simulink model "AGcontrolPIDvelocidadConObsIntegrador_trapPosFinal2017"  (R2017a)
settings: Solver=ode45  StartTime=0.0  StopTime=20  MaxStep=1e-4  RelTol=1e-5  EnableMultiTasking=on
values from neighbouring files (symbols this model uses):
  alfa_cu = 3.9*10^-3    (= 0.0039)    [InicializaYconstantes.m]
  b_m = bm+(bl/r^2)    (= 1.5e-05)    [InicializaYconstantes.m]
  Cts = 1.091    [InicializaYconstantes.m]
  J_m = Jm+(Jl/r^2)    (= 5.65099476805e-06)    [InicializaYconstantes.m]
  Kd = J_m*n*wpos    (= 0.0113019895361)    [InicializaYconstantes.m]
  Ke_int = 3.2768e10    (= 32768000000)    [InicializaYconstantes.m]
  Ketita_corr = 8000    [InicializaYconstantes.m]
  Kew_corr = 25600e3    (= 25600000)    [InicializaYconstantes.m]
  Ki = J_m*wpos^3    (= 2893.30932124)    [InicializaYconstantes.m]
  Kp = J_m*n*wpos^2    (= 9.04159162887)    [InicializaYconstantes.m]
  lambda = 0.01546    [InicializaYconstantes.m]
  Ld = 6.6*10^-3    (= 0.0066)    [InicializaYconstantes.m]
  Lq = 5.8*10^-3    (= 0.0058)    [InicializaYconstantes.m]
  Pp = 3    [InicializaYconstantes.m]
  r = 314.3008    [InicializaYconstantes.m]
  R1 = -p1i*Lq    (= 29)    [InicializaYconstantes.m]
  R2 = -p1i*Ld    (= 33)    [InicializaYconstantes.m]
  Rs = 1.02    [InicializaYconstantes.m]
  Rs_cero = 1.02    [InicializaYconstantes.m]
  Rts = 55    [InicializaYconstantes.m]
  T_l = Tl/r    (= 0.00499521477515)    [InicializaYconstantes.m]
  Ta = 40    [InicializaYconstantes.m]
  Ts0 = 40    [InicializaYconstantes.m]
undefined symbols (not defined in the file or in its folder): sigbuilder_block
libraries: simulink x1
settings Model: Creator=usuario  LastModifiedBy=usuario
settings DataIOCC: LimitDataPoints=on  SaveFormat=Array
settings OptimizationCC: ExpressionDepthLimit=2147483647  LifeSpan=inf
settings DebuggingCC: UnderspecifiedInitializationDetection=Classic  MergeDetectMultiDrivingBlocksExec=none  SolverPrmCheckMsg=warning  StateNameClashWarn=warning  SFUnexpectedBacktrackingDiag=warning  SFNoUnconditionalDefaultTransitionDiag=warning  SFExecutionAtInitializationDiag=none
settings HardwareCC: ProdBitPerPointer=32  ProdBitPerSizeT=32  ProdBitPerPtrDiffT=32  ProdLargestAtomicFloat=None  ProdIntDivRoundTo=Undefined  ProdEndianess=Unspecified  ProdWordSize=32  ProdHWDeviceType=32-bit Generic
settings ModelReferenceCC: PropagateSignalLabelsOutOfModel=off
settings GRTTargetCC: TargetLangStandard=C89/C90 (ANSI)  GeneratePreprocessorConditionals=Disable all
settings ConfigComp: CovMetricSettings=dw  CovHtmlReporting=on  CovSaveCumulativeToWorkspaceVar=on  CovSaveSingleToWorkspaceVar=on  CovExternalEMLEnable=off

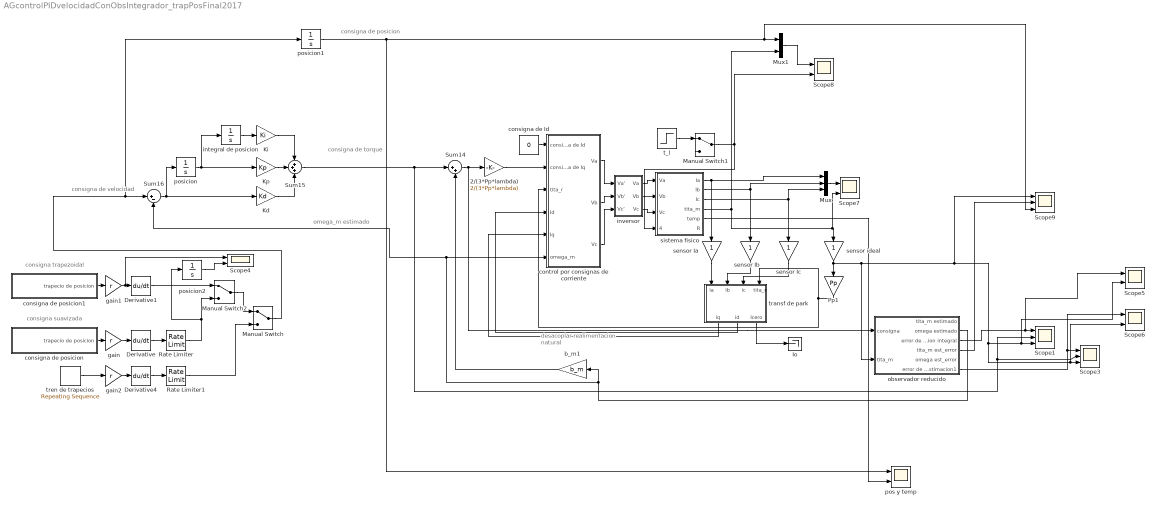
== system AGcontrolPIDvelocidadConObsIntegrador_trapPosFinal2017 ==
  note: consigna trapezoidal
  note: consigna suavizada
  note: consigna de posicion
  note: consigna de velocidad
  note: omega_m estimado
  note: consigna
      | de torque
  note: desacoplar
      | realimentacion natural
  " control por consignas de corriente" : Subsystem
  " pos y temp" : Scope  NumInputPorts=2
  2/(3*Pp*lambda) : Gain  Gain=2/(3*Pp*lambda)
  Derivative : Derivative
  Derivative1 : Derivative
  Derivative4 : Derivative
  Io : Terminator
  Kd : Gain  Gain=Kd
  Ki : Gain  Gain=Ki
  Kp : Gain  Gain=Kp
  Manual Switch : ManualSwitch
  Manual Switch1 : ManualSwitch
  Manual Switch2 : ManualSwitch
  Mux : Mux  Inputs=3
  Mux1 : Mux  Inputs=2
  Pp1 : Gain  Gain=Pp
  Rate Limiter : RateLimiter  RisingSlewLimit=16562  FallingSlewLimit=-16562  SampleTimeMode=inherited
  Rate Limiter1 : RateLimiter  RisingSlewLimit=16562  FallingSlewLimit=-16562  SampleTimeMode=inherited
  Scope1 : Scope  NumInputPorts=3
  Scope3 : Scope  NumInputPorts=3
  Scope{4..8} (5 alike) : Scope  NumInputPorts=2
  Scope9 : Scope  NumInputPorts=3
  Sum14 : Sum  Inputs=|++
  Sum15 : Sum  Inputs=+++
  Sum16 : Sum  Inputs=|+-
  b_m1 : Gain  Gain=b_m
  consigna de Id : Constant  Value=0
  consigna de posicion : Subsystem  Tag=STV Subsys  LoadFcn=sigbuilder_block('load');  StartFcn=sigbuilder_block('start');  StopFcn=sigbuilder_block('stop');  ClipboardFcn=sigbuilder_block('clipboard');  mask(Sigbuilder block){tuvar=[0:10]}
      mask help: Simulink:masks:SigbuilderBlock_MD
      mask init:
      | if ~strcmp(get_param(bdroot(gcbh),'SimulationStatus'),'stopped') tuvar = sigbuilder_block('maskInit'); end
      settings: CopyFcn=sigbuilder_block('copy');  DeleteFcn=sigbuilder_block('delete');  ModelCloseFcn=sigbuilder_block('modelClose');  PreSaveFcn=sigbuilder_block('preSave');  PauseFcn=sigbuilder_block('pause');  ContinueFcn=sigbuilder_block('continue');  NameChangeFcn=sigbuilder_block('namechange');  OpenFcn=sigbuilder_block('open',[5.58621 27.931 836.69 391.034 ]);  CloseFcn=sigbuilder_block('close');
      mask Display: plot(0, 0, 100, 100,[2, 2, 32, 32, 2], [68, 8, 8, 68, 68],[32, 2], [38, 38], [32, 19, 2],[53, 60, 44], [32, 17, 17, 2],[16, 16, 31, 31]);txt = getActiveGroup(gcbh);text(2, 100, txt,'verticalAlignment', 'top');
  consigna de posicion1 : Subsystem  Tag=STV Subsys  LoadFcn=sigbuilder_block('load');  StartFcn=sigbuilder_block('start');  StopFcn=sigbuilder_block('stop');  ClipboardFcn=sigbuilder_block('clipboard');  mask(Sigbuilder block){tuvar=[0:10]}
      mask help: Simulink:masks:SigbuilderBlock_MD
      mask init:
      | if ~strcmp(get_param(bdroot(gcbh),'SimulationStatus'),'stopped') tuvar = sigbuilder_block('maskInit'); end
      settings: CopyFcn=sigbuilder_block('copy');  DeleteFcn=sigbuilder_block('delete');  ModelCloseFcn=sigbuilder_block('modelClose');  PreSaveFcn=sigbuilder_block('preSave');  PauseFcn=sigbuilder_block('pause');  ContinueFcn=sigbuilder_block('continue');  NameChangeFcn=sigbuilder_block('namechange');  OpenFcn=sigbuilder_block('open',[5.58621 27.931 836.69 391.034 ]);  CloseFcn=sigbuilder_block('close');
      mask Display: plot(0, 0, 100, 100,[2, 2, 32, 32, 2], [68, 8, 8, 68, 68],[32, 2], [38, 38], [32, 19, 2],[53, 60, 44], [32, 17, 17, 2],[16, 16, 31, 31]);txt = getActiveGroup(gcbh);text(2, 100, txt,'verticalAlignment', 'top');
  gain : Gain  Gain=r
  gain1 : Gain  Gain=r
  gain2 : Gain  Gain=r
  integral de posicion : Integrator
  inversor : Subsystem
  observador reducido : Subsystem
  posicion : Integrator
  posicion1 : Integrator
  posicion2 : Integrator
  sensor Ia : Gain
  sensor Ib : Gain
  sensor Ic : Gain
  sensor ideal : Gain
  sistema fisico : Subsystem
  t_l : Step  Time=1.1  After=T_l  SampleTime=0
  transf de park : Subsystem
  tren de trapecios : simulink/Sources/Repeating Sequence  rep_seq_t=[0 1 6 11 16 20]  rep_seq_y=[0 0 2*pi 2*pi 0 0]
  wires:
  Ki/1 -> Sum15/1
  Kp/1 -> Sum15/2
  Kd/1 -> Sum15/3
  integral de posicion/1 -> Ki/1
  Sum16/1 -> Kd/1, posicion/1
  sensor Ia/1 -> transf de park/1(ia)
  sensor Ib/1 -> transf de park/2(ib)
  sensor Ic/1 -> transf de park/3(ic)
  inversor/1(Va) -> sistema fisico/1(Va)
  inversor/2(Vb) -> sistema fisico/2(Vb)
  inversor/3(Vc) -> sistema fisico/3(Vc)
  sistema fisico/1(Ia) -> Mux/1, sensor Ia/1
  sistema fisico/2(Ib) -> Mux/2, sensor Ib/1
  sistema fisico/3(Ic) -> Mux/3, sensor Ic/1
  sistema fisico/4(tita_m) -> Mux1/2, Scope7/2, sensor ideal/1
  transf de park/1(iq) -> " control por consignas de corriente"/5(Iq)
  transf de park/3(Icero) -> Io/1
  " control por consignas de corriente"/1(Va) -> inversor/1(Va')
  " control por consignas de corriente"/3(Vc) -> inversor/3(Vc')
  " control por consignas de corriente"/2(Vb) -> inversor/2(Vb')
  consigna de Id/1 -> " control por consignas de corriente"/1(consigna de Id)
  2/(3*Pp*lambda)/1 -> " control por consignas de corriente"/2(consigna de Iq)
  transf de park/2(id) -> " control por consignas de corriente"/4(Id)
  b_m1/1 -> Sum14/2
  Sum14/1 -> observador reducido/1(consigna), 2/(3*Pp*lambda)/1
  posicion/1 -> integral de posicion/1, Kp/1
  Pp1/1 -> transf de park/4(tita_r), " control por consignas de corriente"/3(tita_r)
  Sum15/1 -> Scope3/2, Scope1/2, Sum14/1
  Manual Switch1/1 -> Scope8/2, sistema fisico/4(perturbacion)
  t_l/1 -> Manual Switch1/1
  consigna de posicion/1(trapecio de posicion) -> gain/1
  gain/1 -> Derivative/1
  gain2/1 -> Derivative4/1
  Derivative4/1 -> Rate Limiter1/1
  tren de trapecios/1 -> gain2/1
  Manual Switch/1 -> posicion1/1, Sum16/1
  Rate Limiter1/1 -> Manual Switch/2
  Derivative/1 -> Rate Limiter/1
  sensor ideal/1 -> Scope9/1, Scope5/2, Scope1/3, Scope6/2, Scope3/3, observador reducido/2(tita_m), Pp1/1
  observador reducido/2(omega estimado) -> b_m1/1, Sum16/2, " control por consignas de corriente"/6(omega_m)
  observador reducido/3(error de estimacion integral) -> Scope5/1, Scope1/1
  observador reducido/6(error de estimacion1) -> Scope6/1, Scope3/1
  Mux/1 -> Scope7/1
  Mux1/1 -> Scope8/1
  sistema fisico/5(temp) -> " pos y temp"/2
  posicion1/1 -> " pos y temp"/1, Scope9/3, Mux1/1
  Derivative1/1 -> Manual Switch2/1
  consigna de posicion1/1(trapecio de posicion) -> gain1/1
  gain1/1 -> Scope4/1, Derivative1/1
  Rate Limiter/1 -> posicion2/1, Manual Switch2/2
  Manual Switch2/1 -> Manual Switch/1
  posicion2/1 -> Scope4/2
  observador reducido/4(tita_m est_error) -> Scope9/2

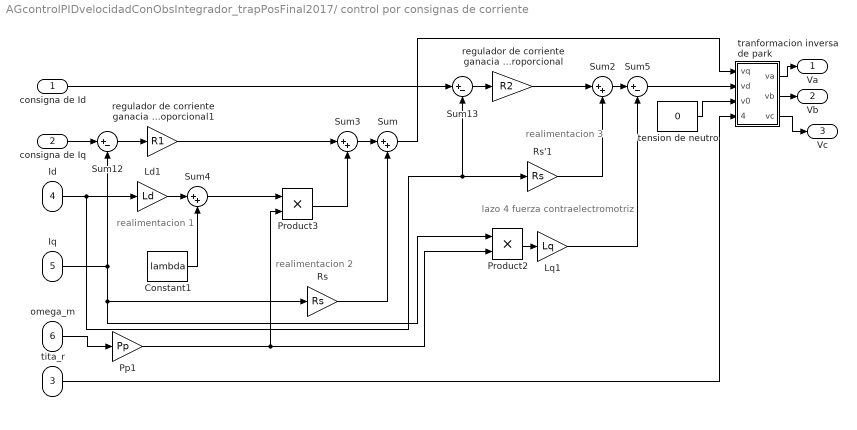
== system AGcontrolPIDvelocidadConObsIntegrador_trapPosFinal2017/ control por consignas de corriente ==
  note: realimentacion 3
  note: realimentacion 1
  note: realimentacion 2
  note: lazo 4 fuerza contraelectromotriz
  consigna de Id : Inport
  consigna de Iq : Inport  Port=2
  tita_r : Inport  Port=3
  Id : Inport  Port=4
  Iq : Inport  Port=5
  omega_m : Inport  Port=6
  Constant1 : Constant  Value=lambda
  Ld1 : Gain  Gain=Ld
  Lq1 : Gain  Gain=Lq
  Pp1 : Gain  Gain=Pp
  Product2 : Product  RndMeth=Zero
  Product3 : Product  RndMeth=Zero
  Rs : Gain  Gain=Rs
  Rs'1 : Gain  Gain=Rs
  Sum{,2..4} (4 alike) : Sum  Inputs=|++
  Sum12 : Sum  Inputs=|+-
  Sum13 : Sum  Inputs=|+-
  Sum5 : Sum  Inputs=|+-
  regulador de corriente ganacia proporcional : Gain  Gain=R2
  regulador de corriente ganacia proporcional1 : Gain  Gain=R1
  tension de neutro : Constant  Value=0
  tranformacion inversa de park : Subsystem
  Va : Outport
  Vb : Outport  Port=2
  Vc : Outport  Port=3
  wires:
  regulador de corriente ganacia proporcional1/1 -> Sum3/1
  tension de neutro/1 -> tranformacion inversa de park/3(v0)
  Rs/1 -> Sum/2
  Constant1/1 -> Sum4/2
  Sum12/1 -> regulador de corriente ganacia proporcional1/1
  Sum5/1 -> tranformacion inversa de park/2(vd)
  tranformacion inversa de park/1(va) -> Va/1
  tranformacion inversa de park/3(vc) -> Vc/1
  Ld1/1 -> Sum4/1
  Sum/1 -> tranformacion inversa de park/1(vq)
  Id/1 -> Ld1/1, Sum13/2, Rs'1/1
  Sum4/1 -> Product3/1
  regulador de corriente ganacia proporcional/1 -> Sum2/1
  consigna de Id/1 -> Sum13/1
  Rs'1/1 -> Sum2/2
  consigna de Iq/1 -> Sum12/1
  tranformacion inversa de park/2(vb) -> Vb/1
  Sum13/1 -> regulador de corriente ganacia proporcional/1
  Product3/1 -> Sum3/2
  Sum3/1 -> Sum/1
  tita_r/1 -> tranformacion inversa de park/4(tita_r)
  Product2/1 -> Lq1/1
  Iq/1 -> Product2/1, Rs/1, Sum12/2
  Lq1/1 -> Sum5/2
  omega_m/1 -> Pp1/1
  Sum2/1 -> Sum5/1
  Pp1/1 -> Product2/2, Product3/2

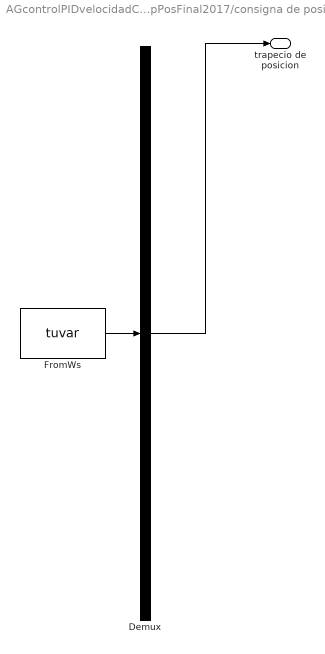
== system AGcontrolPIDvelocidadConObsIntegrador_trapPosFinal2017/consigna de posicion ==
  Demux : Demux  Tag=STV Demux  Outputs=1
  FromWs : FromWorkspace  Tag=STV FromWs  VariableName=tuvar  SampleTime=0
      SigBuilderData=|
      | common.afterFinalStr = 'Extrapolate'
      | common.sampleTime = 0
      | dataSet.timeRange = [0 30]
      | dataSet.name = 'Group 1'
      | sbobj.Groups.Name = 'Group 1'
      | sbobj.Groups.Signals.Name = 'trapecio de posicion'
      | sbobj.Groups.Signals.XData = [0 1 6 11 16 30]
      | sbobj.Groups.Signals.YData = [0 0 6.28318530718 6.28318530718 0 0]
      | sbobj.Groups.TimeRange = [0 30]
  trapecio de posicion : Outport  Tag=STV Outport
  wires:
  Demux/1 -> trapecio de posicion/1
  FromWs/1 -> Demux/1

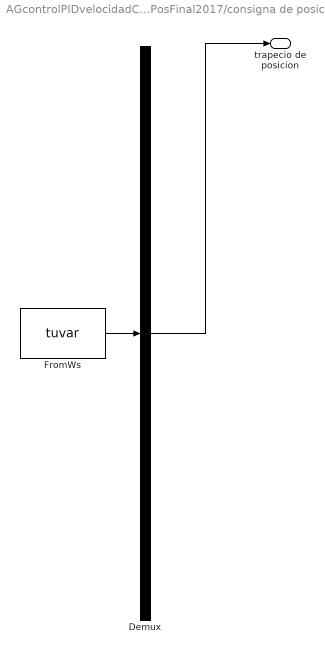
== system AGcontrolPIDvelocidadConObsIntegrador_trapPosFinal2017/consigna de posicion1 ==
  Demux : Demux  Tag=STV Demux  Outputs=1
  FromWs : FromWorkspace  Tag=STV FromWs  VariableName=tuvar  SampleTime=0
      SigBuilderData=|
      | common.afterFinalStr = 'Extrapolate'
      | common.sampleTime = 0
      | dataSet.timeRange = [0 30]
      | dataSet.name = 'Group 1'
      | sbobj.Groups.Name = 'Group 1'
      | sbobj.Groups.Signals.Name = 'trapecio de posicion'
      | sbobj.Groups.Signals.XData = [0 1 6 11 16 30]
      | sbobj.Groups.Signals.YData = [0 0 6.28318530718 6.28318530718 0 0]
      | sbobj.Groups.TimeRange = [0 30]
  trapecio de posicion : Outport  Tag=STV Outport
  wires:
  Demux/1 -> trapecio de posicion/1
  FromWs/1 -> Demux/1

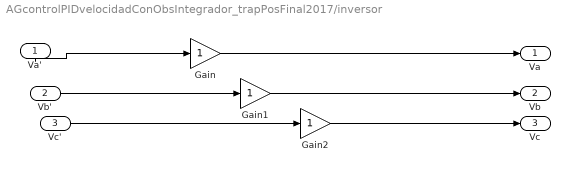
== system AGcontrolPIDvelocidadConObsIntegrador_trapPosFinal2017/inversor ==
  Va' : Inport
  Vb' : Inport  Port=2
  Vc' : Inport  Port=3
  Gain : Gain
  Gain1 : Gain
  Gain2 : Gain
  Va : Outport
  Vb : Outport  Port=2
  Vc : Outport  Port=3
  wires:
  Gain/1 -> Va/1
  Gain1/1 -> Vb/1
  Vb'/1 -> Gain1/1
  Va'/1 -> Gain/1
  Vc'/1 -> Gain2/1
  Gain2/1 -> Vc/1

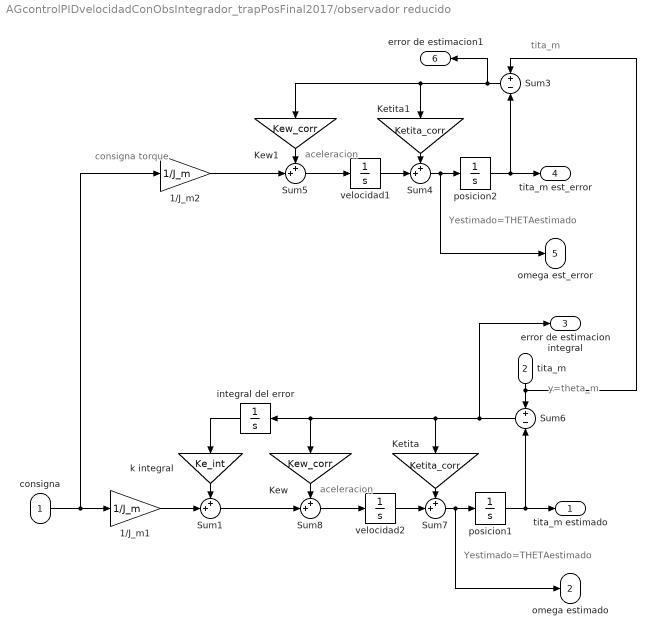
== system AGcontrolPIDvelocidadConObsIntegrador_trapPosFinal2017/observador reducido ==
  note: tita_m
  note: consigna
      | torque
  note: aceleracion
  note: Yestimado=THETAestimado
  note: y=theta_m
  note: Yestimado=THETAestimado
  note: aceleracion
  consigna : Inport
  tita_m : Inport  Port=2
  1/J_m1 : Gain  Gain=1/J_m
  1/J_m2 : Gain  Gain=1/J_m
  Ketita : Gain  Gain=Ketita_corr
  Ketita1 : Gain  Gain=Ketita_corr
  Kew : Gain  Gain=Kew_corr
  Kew1 : Gain  Gain=Kew_corr
  Sum{1,4..5,7..8} (5 alike) : Sum  Inputs=++|
  Sum3 : Sum  Inputs=+-
  Sum6 : Sum  Inputs=+-
  integral del error : Integrator
  k integral : Gain  Gain=Ke_int
  posicion1 : Integrator
  posicion2 : Integrator
  velocidad1 : Integrator
  velocidad2 : Integrator
  tita_m estimado : Outport
  omega estimado : Outport  Port=2
  error de estimacion integral : Outport  Port=3
  tita_m est_error : Outport  Port=4
  omega est_error : Outport  Port=5
  error de estimacion1 : Outport  Port=6
  wires:
  Sum8/1 -> velocidad2/1
  Sum1/1 -> Sum8/2
  Sum7/1 -> omega estimado/1, posicion1/1
  k integral/1 -> Sum1/1
  Kew/1 -> Sum8/1
  posicion1/1 -> tita_m estimado/1, Sum6/2
  1/J_m1/1 -> Sum1/2
  Ketita/1 -> Sum7/1
  velocidad2/1 -> Sum7/2
  integral del error/1 -> k integral/1
  Sum6/1 -> error de estimacion integral/1, Kew/1, integral del error/1, Ketita/1
  Sum4/1 -> omega est_error/1, posicion2/1
  posicion2/1 -> tita_m est_error/1, Sum3/2
  Sum3/1 -> Kew1/1, Ketita1/1, error de estimacion1/1
  Ketita1/1 -> Sum4/1
  Kew1/1 -> Sum5/1
  consigna/1 -> 1/J_m2/1, 1/J_m1/1
  velocidad1/1 -> Sum4/2
  1/J_m2/1 -> Sum5/2
  tita_m/1 -> Sum3/1, Sum6/1
  Sum5/1 -> velocidad1/1

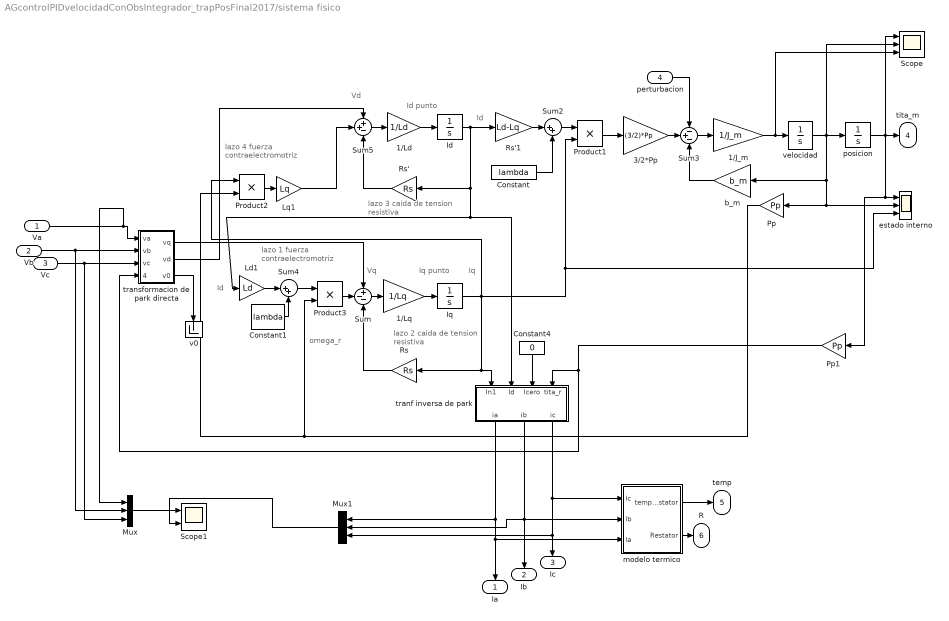
== system AGcontrolPIDvelocidadConObsIntegrador_trapPosFinal2017/sistema fisico ==
  note: Id
  note: lazo 4 fuerza
      |  contraelectromotriz
  note: lazo 3 caida de
      |  tension resistiva
  note: lazo 2 caida de
      |  tension resistiva
  note: lazo 1 fuerza
      |  contraelectromotriz
  note: Vd
  note: Iq
  note: Id punto
  note: Vq
  note: Iq punto
  note: Id
  note: omega_r
  Va : Inport
  Vb : Inport  Port=2
  Vc : Inport  Port=3
  perturbacion : Inport  Port=4
  1/J_m : Gain  Gain=1/J_m
  1/Ld : Gain  Gain=1/Ld
  1/Lq : Gain  Gain=1/Lq
  3/2*Pp : Gain  Gain=(3/2)*Pp
  Constant : Constant  Value=lambda
  Constant1 : Constant  Value=lambda
  Constant4 : Constant  Value=0
  Id : Integrator
  Iq : Integrator
  Ld1 : Gain  Gain=Ld
  Lq1 : Gain  Gain=Lq
  Mux : Mux  Inputs=3
  Mux1 : Mux  Inputs=3
  Pp : Gain  Gain=Pp
  Pp1 : Gain  Gain=Pp
  Product1 : Product  RndMeth=Zero
  Product2 : Product  RndMeth=Zero
  Product3 : Product  RndMeth=Zero
  Rs : Gain  Gain=Rs
  Rs' : Gain  Gain=Rs
  Rs'1 : Gain  Gain=Ld-Lq
  Scope : Scope  NumInputPorts=3
  Scope1 : Scope  NumInputPorts=2
  Sum : Sum  Inputs=+--
  Sum2 : Sum  Inputs=|++
  Sum3 : Sum  Inputs=-+-
  Sum4 : Sum  Inputs=|++
  Sum5 : Sum  Inputs=++-
  b_m : Gain  Gain=b_m
  estado interno : Scope  NumInputPorts=3
  modelo termico : Subsystem
  posicion : Integrator
  "tranf inversa de park " : Subsystem
  transformacion de park directa : Subsystem
  v0 : Terminator
  velocidad : Integrator  ContinuousStateAttributes='velocidad'
  Ia : Outport
  Ib : Outport  Port=2
  Ic : Outport  Port=3
  tita_m : Outport  Port=4
  temp : Outport  Port=5
  R : Outport  Port=6
  wires:
  Constant/1 -> Sum2/2
  Sum2/1 -> Product1/1
  1/Lq/1 -> Iq/1
  Product1/1 -> 3/2*Pp/1
  Ld1/1 -> Sum4/1
  Sum3/1 -> 1/J_m/1
  1/Ld/1 -> Id/1
  Constant1/1 -> Sum4/2
  b_m/1 -> Sum3/3
  Sum/1 -> 1/Lq/1
  Rs/1 -> Sum/3
  perturbacion/1 -> Sum3/1
  Rs'/1 -> Sum5/3
  Product2/1 -> Lq1/1
  Iq/1 -> Rs/1, "tranf inversa de park "/1(In1), Product2/1, Product1/2, estado interno/3
  Product3/1 -> Sum/2
  transformacion de park directa/1(vq) -> Sum/1
  transformacion de park directa/2(vd) -> Sum5/1
  Sum5/1 -> 1/Ld/1
  3/2*Pp/1 -> Sum3/2
  1/J_m/1 -> Scope/3, velocidad/1
  Lq1/1 -> Sum5/2
  transformacion de park directa/3(v0) -> v0/1
  Sum4/1 -> Product3/1
  Id/1 -> Rs'1/1, Rs'/1, "tranf inversa de park "/2(Id), Ld1/1
  Constant4/1 -> "tranf inversa de park "/3(Icero)
  Vc/1 -> Mux/3, transformacion de park directa/3(vc)
  Vb/1 -> Mux/2, transformacion de park directa/2(vb)
  Va/1 -> Mux/1, transformacion de park directa/1(va)
  "tranf inversa de park "/1(ia) -> Mux1/1, modelo termico/3(Ia), Ia/1
  "tranf inversa de park "/2(ib) -> Mux1/2, modelo termico/2(Ib), Ib/1
  "tranf inversa de park "/3(ic) -> modelo termico/1(Ic), Ic/1, Mux1/3
  velocidad/1 -> Scope/2, posicion/1, estado interno/2, Pp/1, b_m/1
  modelo termico/1(tempEstator) -> temp/1
  modelo termico/2(Restator) -> R/1
  Pp/1 -> Product2/2, Product3/2
  posicion/1 -> Scope/1, tita_m/1, estado interno/1, Pp1/1
  Pp1/1 -> transformacion de park directa/4(tita_r), "tranf inversa de park "/4(tita_r)
  Rs'1/1 -> Sum2/1
  Mux/1 -> Scope1/1
  Mux1/1 -> Scope1/2

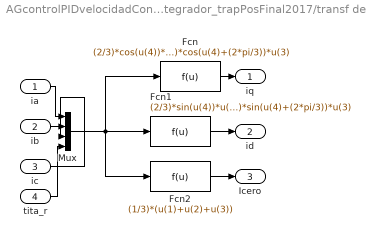
== system AGcontrolPIDvelocidadConObsIntegrador_trapPosFinal2017/transf de park ==
  ia : Inport
  ib : Inport  Port=2
  ic : Inport  Port=3
  tita_r : Inport  Port=4
  Fcn : Fcn  Expr=(2/3)*cos(u(4))*u(1)+(2/3)*cos(u(4)-(2*pi/3))*u(2)+(2/3)*cos(u(4)+(2*pi/3))*u(3)
  Fcn1 : Fcn  Expr=(2/3)*sin(u(4))*u(1)+(2/3)*sin(u(4)-(2*pi/3))*u(2)+(2/3)*sin(u(4)+(2*pi/3))*u(3)
  Fcn2 : Fcn  Expr=(1/3)*(u(1)+u(2)+u(3))
  Mux : Mux
  iq : Outport
  id : Outport  Port=2
  Icero : Outport  Port=3
  wires:
  Mux/1 -> Fcn1/1, Fcn/1, Fcn2/1
  Fcn/1 -> iq/1
  ia/1 -> Mux/1
  ib/1 -> Mux/2
  Fcn1/1 -> id/1
  ic/1 -> Mux/3
  tita_r/1 -> Mux/4
  Fcn2/1 -> Icero/1

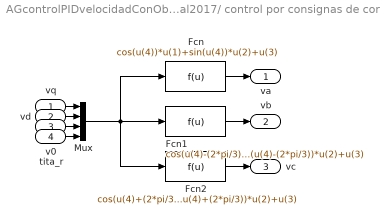
== system AGcontrolPIDvelocidadConObsIntegrador_trapPosFinal2017/ control por consignas de corriente/tranformacion inversa de park ==
  vq : Inport
  vd : Inport  Port=2
  v0 : Inport  Port=3
  tita_r : Inport  Port=4
  Fcn : Fcn  Expr=cos(u(4))*u(1)+sin(u(4))*u(2)+u(3)
  Fcn1 : Fcn  Expr=cos(u(4)-(2*pi/3))*u(1)+sin(u(4)-(2*pi/3))*u(2)+u(3)
  Fcn2 : Fcn  Expr=cos(u(4)+(2*pi/3))*u(1)+sin(u(4)+(2*pi/3))*u(2)+u(3)
  Mux : Mux
  va : Outport
  vb : Outport  Port=2
  vc : Outport  Port=3
  wires:
  Mux/1 -> Fcn1/1, Fcn/1, Fcn2/1
  Fcn/1 -> va/1
  vq/1 -> Mux/1
  vd/1 -> Mux/2
  Fcn1/1 -> vb/1
  v0/1 -> Mux/3
  tita_r/1 -> Mux/4
  Fcn2/1 -> vc/1

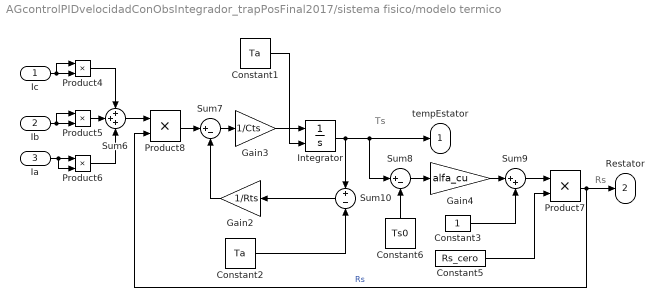
== system AGcontrolPIDvelocidadConObsIntegrador_trapPosFinal2017/sistema fisico/modelo termico ==
  note: Ts
  note: Rs
  Ic : Inport
  Ib : Inport  Port=2
  Ia : Inport  Port=3
  Constant1 : Constant  Value=Ta
  Constant2 : Constant  Value=Ta
  Constant3 : Constant
  Constant5 : Constant  Value=Rs_cero
  Constant6 : Constant  Value=Ts0
  Gain2 : Gain  Gain=1/Rts
  Gain3 : Gain  Gain=1/Cts
  Gain4 : Gain  Gain=alfa_cu
  Integrator : Integrator  InitialConditionSource=external
  Product{4..8} (5 alike) : Product  RndMeth=Zero
  Sum10 : Sum  Inputs=+-
  Sum6 : Sum  Inputs=+++
  Sum7 : Sum  Inputs=|+-
  Sum8 : Sum  Inputs=|+-
  Sum9 : Sum  Inputs=|++
  tempEstator : Outport
  Restator : Outport  Port=2
  wires:
  Gain2/1 -> Sum7/2
  Product4/1 -> Sum6/1
  Gain4/1 -> Sum9/1
  Product6/1 -> Sum6/3
  Gain3/1 -> Integrator/1
  Sum7/1 -> Gain3/1
  Product7/1 -> Product8/2, Restator/1  "Rs"
  Integrator/1 -> Sum10/1, Sum8/1, tempEstator/1
  Constant5/1 -> Product7/2
  Sum9/1 -> Product7/1
  Sum8/1 -> Gain4/1
  Constant3/1 -> Sum9/2
  Sum6/1 -> Product8/1
  Product5/1 -> Sum6/2
  Constant6/1 -> Sum8/2
  Constant2/1 -> Sum10/2
  Product8/1 -> Sum7/1
  Sum10/1 -> Gain2/1
  Ib/1 -> Product5/1, Product5/2
  Ia/1 -> Product6/2, Product6/1
  Ic/1 -> Product4/1, Product4/2
  Constant1/1 -> Integrator/2

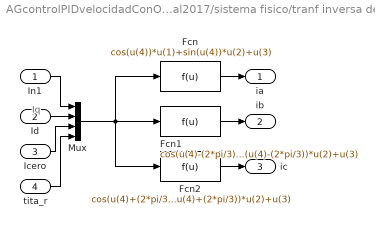
== system AGcontrolPIDvelocidadConObsIntegrador_trapPosFinal2017/sistema fisico/tranf inversa de park  ==
  note: Iq
  In1 : Inport
  Id : Inport  Port=2
  Icero : Inport  Port=3
  tita_r : Inport  Port=4
  Fcn : Fcn  Expr=cos(u(4))*u(1)+sin(u(4))*u(2)+u(3)
  Fcn1 : Fcn  Expr=cos(u(4)-(2*pi/3))*u(1)+sin(u(4)-(2*pi/3))*u(2)+u(3)
  Fcn2 : Fcn  Expr=cos(u(4)+(2*pi/3))*u(1)+sin(u(4)+(2*pi/3))*u(2)+u(3)
  Mux : Mux
  ia : Outport
  ib : Outport  Port=2
  ic : Outport  Port=3
  wires:
  Mux/1 -> Fcn1/1, Fcn/1, Fcn2/1
  Fcn/1 -> ia/1
  In1/1 -> Mux/1
  Id/1 -> Mux/2
  Fcn1/1 -> ib/1
  Icero/1 -> Mux/3
  tita_r/1 -> Mux/4
  Fcn2/1 -> ic/1

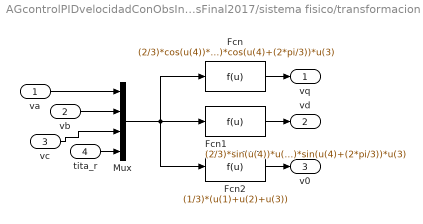
== system AGcontrolPIDvelocidadConObsIntegrador_trapPosFinal2017/sistema fisico/transformacion de park directa ==
  va : Inport
  vb : Inport  Port=2
  vc : Inport  Port=3
  tita_r : Inport  Port=4
  Fcn : Fcn  Expr=(2/3)*cos(u(4))*u(1)+(2/3)*cos(u(4)-(2*pi/3))*u(2)+(2/3)*cos(u(4)+(2*pi/3))*u(3)
  Fcn1 : Fcn  Expr=(2/3)*sin(u(4))*u(1)+(2/3)*sin(u(4)-(2*pi/3))*u(2)+(2/3)*sin(u(4)+(2*pi/3))*u(3)
  Fcn2 : Fcn  Expr=(1/3)*(u(1)+u(2)+u(3))
  Mux : Mux
  vq : Outport
  vd : Outport  Port=2
  v0 : Outport  Port=3
  wires:
  Mux/1 -> Fcn2/1, Fcn1/1, Fcn/1
  Fcn/1 -> vq/1
  va/1 -> Mux/1
  vb/1 -> Mux/2
  Fcn1/1 -> vd/1
  vc/1 -> Mux/3
  tita_r/1 -> Mux/4
  Fcn2/1 -> v0/1
